simulink model "Test_Decoder_3_to_8"  (Simulink 8.1)
settings: Solver=ode45  StartTime=0.0  StopTime=len  RelTol=1e-3
libraries: commutil2 x2, Decoders_Lib x1
settings Model: Creator=N  LastModifiedBy=uzivatel
settings DataIOCC: LimitDataPoints=off  SignalLoggingSaveFormat=Dataset
settings OptimizationCC: ExpressionDepthLimit=128
settings DebuggingCC: UnderspecifiedInitializationDetection=Simplified  MergeDetectMultiDrivingBlocksExec=error  SolverPrmCheckMsg=none  FcnCallInpInsideContextMsg=EnableAllAsError  FrameProcessingCompatibilityMsg=error  StateNameClashWarn=none
settings HardwareCC: ProdBitPerPointer=64  ProdLargestAtomicFloat=Float  ProdIntDivRoundTo=Zero  ProdEndianess=LittleEndian  ProdHWDeviceType=Intel->x86-64 (Windows64)
settings ModelReferenceCC: PropagateSignalLabelsOutOfModel=on
settings GRTTargetCC: CodeReplacementLibrary=None  CombineOutputUpdateFcns=on  CPPClassGenCompliant=on  GRTInterface=off

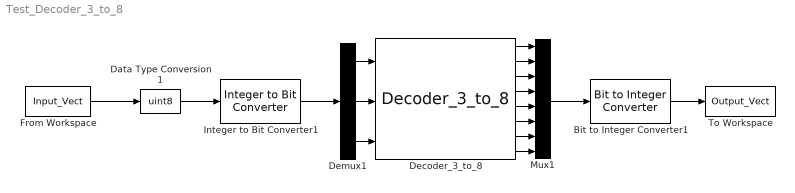
== system Test_Decoder_3_to_8 ==
  Bit to Integer Converter1 : commutil2/Bit to Integer Converter  nbits=8  bitOrder=MSB first  signedOutputValues=Unsigned  outDtype=uint8  outDtypeSigned=Inherit via internal rule
  Data Type Conversion1 : DataTypeConversion  OutDataTypeStr=uint8
  Decoder_3_to_8 : Decoders_Lib/Decoders_Lib/Decoder_3_to_8
  Demux1 : Demux  Outputs=3
  From Workspace : FromWorkspace  VariableName=Input_Vect  SampleTime=1  Interpolate=off  OutputAfterFinalValue=Holding final value
  Integer to Bit Converter1 : commutil2/Integer to Bit Converter  nbits=3  signedInputValues=Unsigned  bitOrder=MSB first  outDtype=uint8
  Mux1 : Mux  Inputs=8
  To Workspace : ToWorkspace  VariableName=Output_Vect  SampleTime=1
  wires:
  Decoder_3_to_8/1 -> Mux1/1
  Decoder_3_to_8/8 -> Mux1/8
  Decoder_3_to_8/7 -> Mux1/7
  Decoder_3_to_8/6 -> Mux1/6
  Decoder_3_to_8/5 -> Mux1/5
  Decoder_3_to_8/4 -> Mux1/4
  Decoder_3_to_8/3 -> Mux1/3
  Decoder_3_to_8/2 -> Mux1/2
  Mux1/1 -> Bit to Integer Converter1/1
  Demux1/2 -> Decoder_3_to_8/2
  Demux1/3 -> Decoder_3_to_8/3
  Demux1/1 -> Decoder_3_to_8/1
  Integer to Bit Converter1/1 -> Demux1/1
  Data Type Conversion1/1 -> Integer to Bit Converter1/1
  From Workspace/1 -> Data Type Conversion1/1
  Bit to Integer Converter1/1 -> To Workspace/1
